simulink model "EEBL_Scenario_01_cs"  (Simulink 7.6)
settings: Solver=ode5  SolverMode=SingleTasking  StartTime=0.0  StopTime=inf  FixedStep=1/100  RelTol=1e-3
PreLoadFcn:
  | check_NUTS_defined;
  | 
  | assignin('base',['model_closed_' bdroot],false);addpath('../includes_V2x');
InitFcn:
  | PreScanExperimentInitFcn(bdroot)
StopFcn:
  | PreScanExperimentStopFcn(bdroot)
undefined symbols (not defined in the file or in its folder): acceleration, actorID, actorType, DiscIntNeverNeededParam, GPS_alt, GPS_lat, GPS_long, intmax, lightBarInUse, messageID, publicVehicleType, rotZ, sireneInUse, trafficLightPriority, turnAdvice, velocity, x_ini_VRML, y_ini_VRML, yawRate, z_ini_VRML
libraries: simulink x58, PreScanSimulinkLibrary x12, simulink_extras x10, PreScanUsefulBlocks x6, simulink_need_slupdate x1
(part 5 of 10)

== system EEBL_Scenario_01_cs/BMW_X5_1/Antenna_Rx_3_Demux ==
  AntennaR : Inport
  Bus Creator : BusCreator  Inputs=200
  Demux : Demux  Outputs=228
  Demux1 : Demux  Outputs=3
  Mux : Mux  Inputs=3
  Reorder : Subsystem  mask(Output reorder block){NrOfOutputs=228, NrOfObjects=2}
      mask prompts: NrOfOutputs "Number Of Outputs [-]"; NrOfObjects "Number Of Objects [-]"
      mask help: Change output order from object based to output type based
      mask init: same as EEBL_Scenario_01_cs/Audi_A8_1/Antenna_Rx_1_Demux/Reorder
  Terminator_{9..12,17..18,20..23,25..30} (16 alike) : Terminator
  compas converter : Subsystem
  xyz2GPS : PreScanUsefulBlocks/xyz2GPS  CoordinateCount=2  GPS_base=[0.000000 0.000000 0.000]
  Vehicle_ID : Outport
  GPS_pos_lat_[deg] : Outport  Port=2
  GPS_pos_long_[deg] : Outport  Port=3
  GPS_pos_alt_[m] : Outport  Port=4
  Velocity_[m/s] : Outport  Port=5
  Acceleration_[m/s2] : Outport  Port=6
  Heading [deg] : Outport  Port=7
  warning_signal_id : Outport  Port=8
  maneuvre_id : Outport  Port=9
  vehicle_type : Outport  Port=10
  brakingcapacity : Outport  Port=11
  vehicle_size : Outport  Port=12
  spare : Outport  Port=13
  wires:
  Bus Creator/1 -> spare/1
  compas converter/1(heading [deg]) -> Heading [deg]/1
  Demux/1 -> Vehicle_ID/1
  Demux/2 -> Terminator_9/1
  Demux/3 -> Terminator_10/1
  Demux/4 -> Terminator_11/1
  Demux/5 -> Terminator_12/1
  Demux/6 -> Mux/1  "pos_x"
  Demux/7 -> Mux/2  "pos_y"
  Demux/8 -> Mux/3  "pos_z"
  Demux/10 -> Terminator_17/1
  Demux/11 -> Terminator_18/1
  Demux/12 -> Acceleration_[m/s2]/1
  Demux/13 -> Terminator_20/1
  Demux/14 -> Terminator_21/1
  Demux/15 -> Terminator_22/1
  Demux/16 -> Terminator_23/1
  Demux/17 -> compas converter/1(rotz [rad])
  Demux/18 -> Terminator_25/1
  Demux/19 -> Terminator_26/1
  Demux/20 -> Terminator_27/1
  Demux/21 -> Terminator_28/1
  Demux/22 -> Terminator_29/1
  Demux/23 -> Terminator_30/1
  Demux/9 -> Velocity_[m/s]/1
  Demux/24 -> warning_signal_id/1
  Demux/25 -> maneuvre_id/1
  Demux/26 -> vehicle_type/1
  Demux/27 -> brakingcapacity/1
  Demux/28 -> vehicle_size/1
  xyz2GPS/1 -> Demux1/1
  Demux1/1 -> GPS_pos_lat_[deg]/1
  Demux1/2 -> GPS_pos_long_[deg]/1
  Demux1/3 -> GPS_pos_alt_[m]/1
  Mux/1 -> xyz2GPS/1
  Reorder/1(Out) -> Demux/1
  AntennaR/1 -> Reorder/1(In)
  Demux/29 -> Bus Creator/1  "warning"
  Demux/30 -> Bus Creator/2  "messageID"
  Demux/31 -> Bus Creator/3  "actorID"
  Demux/32 -> Bus Creator/4  "actorType"
  Demux/33 -> Bus Creator/5  "publicVehicleType"
  Demux/34 -> Bus Creator/6  "lightBarInUse"
  Demux/35 -> Bus Creator/7  "sireneInUse"
  Demux/36 -> Bus Creator/8  "velocity"
  Demux/37 -> Bus Creator/9  "acceleration"
  Demux/38 -> Bus Creator/10  "yawRate"
  Demux/39 -> Bus Creator/11  "turnAdvice"
  Demux/40 -> Bus Creator/12  "trafficLightPriority"
  Demux/41 -> Bus Creator/13  "GPS_lat"
  Demux/42 -> Bus Creator/14  "GPS_long"
  Demux/43 -> Bus Creator/15  "GPS_alt"
  Demux/44 -> Bus Creator/16  "rotZ"
  Demux/45 -> Bus Creator/17  "spare_17"
  Demux/46 -> Bus Creator/18  "spare_18"
  Demux/47 -> Bus Creator/19  "spare_19"
  Demux/48 -> Bus Creator/20  "spare_20"
  Demux/49 -> Bus Creator/21  "spare_21"
  Demux/50 -> Bus Creator/22  "spare_22"
  Demux/51 -> Bus Creator/23  "spare_23"
  Demux/52 -> Bus Creator/24  "spare_24"
  Demux/53 -> Bus Creator/25  "spare_25"
  Demux/54 -> Bus Creator/26  "spare_26"
  Demux/55 -> Bus Creator/27  "spare_27"
  Demux/56 -> Bus Creator/28  "spare_28"
  Demux/57 -> Bus Creator/29  "spare_29"
  Demux/58 -> Bus Creator/30  "spare_30"
  Demux/59 -> Bus Creator/31  "spare_31"
  Demux/60 -> Bus Creator/32  "spare_32"
  Demux/61 -> Bus Creator/33  "spare_33"
  Demux/62 -> Bus Creator/34  "spare_34"
  Demux/63 -> Bus Creator/35  "spare_35"
  Demux/64 -> Bus Creator/36  "spare_36"
  Demux/65 -> Bus Creator/37  "spare_37"
  Demux/66 -> Bus Creator/38  "spare_38"
  Demux/67 -> Bus Creator/39  "spare_39"
  Demux/68 -> Bus Creator/40  "spare_40"
  Demux/69 -> Bus Creator/41  "spare_41"
  Demux/70 -> Bus Creator/42  "spare_42"
  Demux/71 -> Bus Creator/43  "spare_43"
  Demux/72 -> Bus Creator/44  "spare_44"
  Demux/73 -> Bus Creator/45  "spare_45"
  Demux/74 -> Bus Creator/46  "spare_46"
  Demux/75 -> Bus Creator/47  "spare_47"
  Demux/76 -> Bus Creator/48  "spare_48"
  Demux/77 -> Bus Creator/49  "spare_49"
  Demux/78 -> Bus Creator/50  "spare_50"
  Demux/79 -> Bus Creator/51  "spare_51"
  Demux/80 -> Bus Creator/52  "spare_52"
  Demux/81 -> Bus Creator/53  "spare_53"
  Demux/82 -> Bus Creator/54  "spare_54"
  Demux/83 -> Bus Creator/55  "spare_55"
  Demux/84 -> Bus Creator/56  "spare_56"
  Demux/85 -> Bus Creator/57  "spare_57"
  Demux/86 -> Bus Creator/58  "spare_58"
  Demux/87 -> Bus Creator/59  "spare_59"
  Demux/88 -> Bus Creator/60  "spare_60"
  Demux/89 -> Bus Creator/61  "spare_61"
  Demux/90 -> Bus Creator/62  "spare_62"
  Demux/91 -> Bus Creator/63  "spare_63"
  Demux/92 -> Bus Creator/64  "spare_64"
  Demux/93 -> Bus Creator/65  "spare_65"
  Demux/94 -> Bus Creator/66  "spare_66"
  Demux/95 -> Bus Creator/67  "spare_67"
  Demux/96 -> Bus Creator/68  "spare_68"
  Demux/97 -> Bus Creator/69  "spare_69"
  Demux/98 -> Bus Creator/70  "spare_70"
  Demux/99 -> Bus Creator/71  "spare_71"
  Demux/100 -> Bus Creator/72  "spare_72"
  Demux/101 -> Bus Creator/73  "spare_73"
  Demux/102 -> Bus Creator/74  "spare_74"
  Demux/103 -> Bus Creator/75  "spare_75"
  Demux/104 -> Bus Creator/76  "spare_76"
  Demux/105 -> Bus Creator/77  "spare_77"
  Demux/106 -> Bus Creator/78  "spare_78"
  Demux/107 -> Bus Creator/79  "spare_79"
  Demux/108 -> Bus Creator/80  "spare_80"
  Demux/109 -> Bus Creator/81  "spare_81"
  Demux/110 -> Bus Creator/82  "spare_82"
  Demux/111 -> Bus Creator/83  "spare_83"
  Demux/112 -> Bus Creator/84  "spare_84"
  Demux/113 -> Bus Creator/85  "spare_85"
  Demux/114 -> Bus Creator/86  "spare_86"
  Demux/115 -> Bus Creator/87  "spare_87"
  Demux/116 -> Bus Creator/88  "spare_88"
  Demux/117 -> Bus Creator/89  "spare_89"
  Demux/118 -> Bus Creator/90  "spare_90"
  Demux/119 -> Bus Creator/91  "spare_91"
  Demux/120 -> Bus Creator/92  "spare_92"
  Demux/121 -> Bus Creator/93  "spare_93"
  Demux/122 -> Bus Creator/94  "spare_94"
  Demux/123 -> Bus Creator/95  "spare_95"
  Demux/124 -> Bus Creator/96  "spare_96"
  Demux/125 -> Bus Creator/97  "spare_97"
  Demux/126 -> Bus Creator/98  "spare_98"
  Demux/127 -> Bus Creator/99  "spare_99"
  Demux/128 -> Bus Creator/100  "spare_100"
  Demux/129 -> Bus Creator/101  "spare_101"
  Demux/130 -> Bus Creator/102  "spare_102"
  Demux/131 -> Bus Creator/103  "spare_103"
  Demux/132 -> Bus Creator/104  "spare_104"
  Demux/133 -> Bus Creator/105  "spare_105"
  Demux/134 -> Bus Creator/106  "spare_106"
  Demux/135 -> Bus Creator/107  "spare_107"
  Demux/136 -> Bus Creator/108  "spare_108"
  Demux/137 -> Bus Creator/109  "spare_109"
  Demux/138 -> Bus Creator/110  "spare_110"
  Demux/139 -> Bus Creator/111  "spare_111"
  Demux/140 -> Bus Creator/112  "spare_112"
  Demux/141 -> Bus Creator/113  "spare_113"
  Demux/142 -> Bus Creator/114  "spare_114"
  Demux/143 -> Bus Creator/115  "spare_115"
  Demux/144 -> Bus Creator/116  "spare_116"
  Demux/145 -> Bus Creator/117  "spare_117"
  Demux/146 -> Bus Creator/118  "spare_118"
  Demux/147 -> Bus Creator/119  "spare_119"
  Demux/148 -> Bus Creator/120  "spare_120"
  Demux/149 -> Bus Creator/121  "spare_121"
  Demux/150 -> Bus Creator/122  "spare_122"
  Demux/151 -> Bus Creator/123  "spare_123"
  Demux/152 -> Bus Creator/124  "spare_124"
  Demux/153 -> Bus Creator/125  "spare_125"
  Demux/154 -> Bus Creator/126  "spare_126"
  Demux/155 -> Bus Creator/127  "spare_127"
  Demux/156 -> Bus Creator/128  "spare_128"
  Demux/157 -> Bus Creator/129  "spare_129"
  Demux/158 -> Bus Creator/130  "spare_130"
  Demux/159 -> Bus Creator/131  "spare_131"
  Demux/160 -> Bus Creator/132  "spare_132"
  Demux/161 -> Bus Creator/133  "spare_133"
  Demux/162 -> Bus Creator/134  "spare_134"
  Demux/163 -> Bus Creator/135  "spare_135"
  Demux/164 -> Bus Creator/136  "spare_136"
  Demux/165 -> Bus Creator/137  "spare_137"
  Demux/166 -> Bus Creator/138  "spare_138"
  Demux/167 -> Bus Creator/139  "spare_139"
  Demux/168 -> Bus Creator/140  "spare_140"
  Demux/169 -> Bus Creator/141  "spare_141"
  Demux/170 -> Bus Creator/142  "spare_142"
  Demux/171 -> Bus Creator/143  "spare_143"
  Demux/172 -> Bus Creator/144  "spare_144"
  Demux/173 -> Bus Creator/145  "spare_145"
  Demux/174 -> Bus Creator/146  "spare_146"
  Demux/175 -> Bus Creator/147  "spare_147"
  Demux/176 -> Bus Creator/148  "spare_148"
  Demux/177 -> Bus Creator/149  "spare_149"
  Demux/178 -> Bus Creator/150  "spare_150"
  Demux/179 -> Bus Creator/151  "spare_151"
  Demux/180 -> Bus Creator/152  "spare_152"
  Demux/181 -> Bus Creator/153  "spare_153"
  Demux/182 -> Bus Creator/154  "spare_154"
  Demux/183 -> Bus Creator/155  "spare_155"
  Demux/184 -> Bus Creator/156  "spare_156"
  Demux/185 -> Bus Creator/157  "spare_157"
  Demux/186 -> Bus Creator/158  "spare_158"
  Demux/187 -> Bus Creator/159  "spare_159"
  Demux/188 -> Bus Creator/160  "spare_160"
  Demux/189 -> Bus Creator/161  "spare_161"
  Demux/190 -> Bus Creator/162  "spare_162"
  Demux/191 -> Bus Creator/163  "spare_163"
  Demux/192 -> Bus Creator/164  "spare_164"
  Demux/193 -> Bus Creator/165  "spare_165"
  Demux/194 -> Bus Creator/166  "spare_166"
  Demux/195 -> Bus Creator/167  "spare_167"
  Demux/196 -> Bus Creator/168  "spare_168"
  Demux/197 -> Bus Creator/169  "spare_169"
  Demux/198 -> Bus Creator/170  "spare_170"
  Demux/199 -> Bus Creator/171  "spare_171"
  Demux/200 -> Bus Creator/172  "spare_172"
  Demux/201 -> Bus Creator/173  "spare_173"
  Demux/202 -> Bus Creator/174  "spare_174"
  Demux/203 -> Bus Creator/175  "spare_175"
  Demux/204 -> Bus Creator/176  "spare_176"
  Demux/205 -> Bus Creator/177  "spare_177"
  Demux/206 -> Bus Creator/178  "spare_178"
  Demux/207 -> Bus Creator/179  "spare_179"
  Demux/208 -> Bus Creator/180  "spare_180"
  Demux/209 -> Bus Creator/181  "spare_181"
  Demux/210 -> Bus Creator/182  "spare_182"
  Demux/211 -> Bus Creator/183  "spare_183"
  Demux/212 -> Bus Creator/184  "spare_184"
  Demux/213 -> Bus Creator/185  "spare_185"
  Demux/214 -> Bus Creator/186  "spare_186"
  Demux/215 -> Bus Creator/187  "spare_187"
  Demux/216 -> Bus Creator/188  "spare_188"
  Demux/217 -> Bus Creator/189  "spare_189"
  Demux/218 -> Bus Creator/190  "spare_190"
  Demux/219 -> Bus Creator/191  "spare_191"
  Demux/220 -> Bus Creator/192  "spare_192"
  Demux/221 -> Bus Creator/193  "spare_193"
  Demux/222 -> Bus Creator/194  "spare_194"
  Demux/223 -> Bus Creator/195  "spare_195"
  Demux/224 -> Bus Creator/196  "spare_196"
  Demux/225 -> Bus Creator/197  "spare_197"
  Demux/226 -> Bus Creator/198  "spare_198"
  Demux/227 -> Bus Creator/199  "spare_199"
  Demux/228 -> Bus Creator/200  "spare_200"

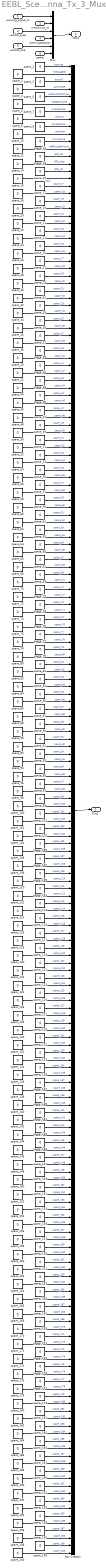
== system EEBL_Scenario_01_cs/BMW_X5_1/Antenna_Tx_3_Mux ==
  warning_signal_id : Inport  SampleTime=TimeStep
  maneuvre_id : Inport  Port=2  SampleTime=TimeStep
  vehicle_type : Inport  Port=3  SampleTime=TimeStep
  brakingcapacity : Inport  Port=4  SampleTime=TimeStep
  vehicle_size : Inport  Port=5  SampleTime=TimeStep
  spare : Inport  Port=6  SampleTime=TimeStep
  Bus Creator : BusCreator  Inputs=200
  Mux : Mux  Inputs=6
  spare_{1..200} (200 alike) : Constant  Value=0  SampleTime=TimeStep
  Out1 : Outport
  Out2 : Outport  Port=2  SampleTime=TimeStep
  wires:
  spare_200/1 -> Bus Creator/200  "spare_200"
  spare_199/1 -> Bus Creator/199  "spare_199"
  spare_198/1 -> Bus Creator/198  "spare_198"
  spare_197/1 -> Bus Creator/197  "spare_197"
  spare_196/1 -> Bus Creator/196  "spare_196"
  spare_195/1 -> Bus Creator/195  "spare_195"
  spare_194/1 -> Bus Creator/194  "spare_194"
  spare_193/1 -> Bus Creator/193  "spare_193"
  spare_192/1 -> Bus Creator/192  "spare_192"
  spare_191/1 -> Bus Creator/191  "spare_191"
  spare_190/1 -> Bus Creator/190  "spare_190"
  spare_189/1 -> Bus Creator/189  "spare_189"
  spare_188/1 -> Bus Creator/188  "spare_188"
  spare_187/1 -> Bus Creator/187  "spare_187"
  spare_186/1 -> Bus Creator/186  "spare_186"
  spare_185/1 -> Bus Creator/185  "spare_185"
  spare_184/1 -> Bus Creator/184  "spare_184"
  spare_183/1 -> Bus Creator/183  "spare_183"
  spare_182/1 -> Bus Creator/182  "spare_182"
  spare_181/1 -> Bus Creator/181  "spare_181"
  spare_180/1 -> Bus Creator/180  "spare_180"
  spare_179/1 -> Bus Creator/179  "spare_179"
  spare_178/1 -> Bus Creator/178  "spare_178"
  spare_177/1 -> Bus Creator/177  "spare_177"
  spare_176/1 -> Bus Creator/176  "spare_176"
  spare_175/1 -> Bus Creator/175  "spare_175"
  spare_174/1 -> Bus Creator/174  "spare_174"
  spare_173/1 -> Bus Creator/173  "spare_173"
  spare_172/1 -> Bus Creator/172  "spare_172"
  spare_171/1 -> Bus Creator/171  "spare_171"
  spare_170/1 -> Bus Creator/170  "spare_170"
  spare_169/1 -> Bus Creator/169  "spare_169"
  spare_168/1 -> Bus Creator/168  "spare_168"
  spare_167/1 -> Bus Creator/167  "spare_167"
  spare_166/1 -> Bus Creator/166  "spare_166"
  spare_165/1 -> Bus Creator/165  "spare_165"
  spare_164/1 -> Bus Creator/164  "spare_164"
  spare_163/1 -> Bus Creator/163  "spare_163"
  spare_162/1 -> Bus Creator/162  "spare_162"
  spare_161/1 -> Bus Creator/161  "spare_161"
  spare_160/1 -> Bus Creator/160  "spare_160"
  spare_159/1 -> Bus Creator/159  "spare_159"
  spare_158/1 -> Bus Creator/158  "spare_158"
  spare_157/1 -> Bus Creator/157  "spare_157"
  spare_156/1 -> Bus Creator/156  "spare_156"
  spare_155/1 -> Bus Creator/155  "spare_155"
  spare_154/1 -> Bus Creator/154  "spare_154"
  spare_153/1 -> Bus Creator/153  "spare_153"
  spare_152/1 -> Bus Creator/152  "spare_152"
  spare_151/1 -> Bus Creator/151  "spare_151"
  spare_150/1 -> Bus Creator/150  "spare_150"
  spare_149/1 -> Bus Creator/149  "spare_149"
  spare_148/1 -> Bus Creator/148  "spare_148"
  spare_147/1 -> Bus Creator/147  "spare_147"
  spare_146/1 -> Bus Creator/146  "spare_146"
  spare_145/1 -> Bus Creator/145  "spare_145"
  spare_144/1 -> Bus Creator/144  "spare_144"
  spare_143/1 -> Bus Creator/143  "spare_143"
  spare_142/1 -> Bus Creator/142  "spare_142"
  spare_141/1 -> Bus Creator/141  "spare_141"
  spare_140/1 -> Bus Creator/140  "spare_140"
  spare_139/1 -> Bus Creator/139  "spare_139"
  spare_138/1 -> Bus Creator/138  "spare_138"
  spare_137/1 -> Bus Creator/137  "spare_137"
  spare_136/1 -> Bus Creator/136  "spare_136"
  spare_135/1 -> Bus Creator/135  "spare_135"
  spare_134/1 -> Bus Creator/134  "spare_134"
  spare_133/1 -> Bus Creator/133  "spare_133"
  spare_132/1 -> Bus Creator/132  "spare_132"
  spare_131/1 -> Bus Creator/131  "spare_131"
  spare_130/1 -> Bus Creator/130  "spare_130"
  spare_129/1 -> Bus Creator/129  "spare_129"
  spare_128/1 -> Bus Creator/128  "spare_128"
  spare_127/1 -> Bus Creator/127  "spare_127"
  spare_126/1 -> Bus Creator/126  "spare_126"
  spare_125/1 -> Bus Creator/125  "spare_125"
  spare_124/1 -> Bus Creator/124  "spare_124"
  spare_123/1 -> Bus Creator/123  "spare_123"
  spare_122/1 -> Bus Creator/122  "spare_122"
  spare_121/1 -> Bus Creator/121  "spare_121"
  spare_120/1 -> Bus Creator/120  "spare_120"
  spare_119/1 -> Bus Creator/119  "spare_119"
  spare_118/1 -> Bus Creator/118  "spare_118"
  spare_117/1 -> Bus Creator/117  "spare_117"
  spare_116/1 -> Bus Creator/116  "spare_116"
  spare_115/1 -> Bus Creator/115  "spare_115"
  spare_114/1 -> Bus Creator/114  "spare_114"
  spare_113/1 -> Bus Creator/113  "spare_113"
  spare_112/1 -> Bus Creator/112  "spare_112"
  spare_111/1 -> Bus Creator/111  "spare_111"
  spare_110/1 -> Bus Creator/110  "spare_110"
  spare_109/1 -> Bus Creator/109  "spare_109"
  spare_108/1 -> Bus Creator/108  "spare_108"
  spare_107/1 -> Bus Creator/107  "spare_107"
  spare_106/1 -> Bus Creator/106  "spare_106"
  spare_105/1 -> Bus Creator/105  "spare_105"
  spare_104/1 -> Bus Creator/104  "spare_104"
  spare_103/1 -> Bus Creator/103  "spare_103"
  spare_102/1 -> Bus Creator/102  "spare_102"
  spare_101/1 -> Bus Creator/101  "spare_101"
  spare_100/1 -> Bus Creator/100  "spare_100"
  spare_99/1 -> Bus Creator/99  "spare_99"
  spare_98/1 -> Bus Creator/98  "spare_98"
  spare_97/1 -> Bus Creator/97  "spare_97"
  spare_96/1 -> Bus Creator/96  "spare_96"
  spare_95/1 -> Bus Creator/95  "spare_95"
  spare_94/1 -> Bus Creator/94  "spare_94"
  spare_93/1 -> Bus Creator/93  "spare_93"
  spare_92/1 -> Bus Creator/92  "spare_92"
  spare_91/1 -> Bus Creator/91  "spare_91"
  spare_90/1 -> Bus Creator/90  "spare_90"
  spare_89/1 -> Bus Creator/89  "spare_89"
  spare_88/1 -> Bus Creator/88  "spare_88"
  spare_87/1 -> Bus Creator/87  "spare_87"
  spare_86/1 -> Bus Creator/86  "spare_86"
  spare_85/1 -> Bus Creator/85  "spare_85"
  spare_84/1 -> Bus Creator/84  "spare_84"
  spare_83/1 -> Bus Creator/83  "spare_83"
  spare_82/1 -> Bus Creator/82  "spare_82"
  spare_81/1 -> Bus Creator/81  "spare_81"
  spare_80/1 -> Bus Creator/80  "spare_80"
  spare_79/1 -> Bus Creator/79  "spare_79"
  spare_78/1 -> Bus Creator/78  "spare_78"
  spare_77/1 -> Bus Creator/77  "spare_77"
  spare_76/1 -> Bus Creator/76  "spare_76"
  spare_75/1 -> Bus Creator/75  "spare_75"
  spare_74/1 -> Bus Creator/74  "spare_74"
  spare_73/1 -> Bus Creator/73  "spare_73"
  spare_72/1 -> Bus Creator/72  "spare_72"
  spare_71/1 -> Bus Creator/71  "spare_71"
  spare_70/1 -> Bus Creator/70  "spare_70"
  spare_69/1 -> Bus Creator/69  "spare_69"
  spare_68/1 -> Bus Creator/68  "spare_68"
  spare_67/1 -> Bus Creator/67  "spare_67"
  spare_66/1 -> Bus Creator/66  "spare_66"
  spare_65/1 -> Bus Creator/65  "spare_65"
  spare_64/1 -> Bus Creator/64  "spare_64"
  spare_63/1 -> Bus Creator/63  "spare_63"
  spare_62/1 -> Bus Creator/62  "spare_62"
  spare_61/1 -> Bus Creator/61  "spare_61"
  spare_60/1 -> Bus Creator/60  "spare_60"
  spare_59/1 -> Bus Creator/59  "spare_59"
  spare_58/1 -> Bus Creator/58  "spare_58"
  spare_57/1 -> Bus Creator/57  "spare_57"
  spare_56/1 -> Bus Creator/56  "spare_56"
  spare_55/1 -> Bus Creator/55  "spare_55"
  spare_54/1 -> Bus Creator/54  "spare_54"
  spare_53/1 -> Bus Creator/53  "spare_53"
  spare_52/1 -> Bus Creator/52  "spare_52"
  spare_51/1 -> Bus Creator/51  "spare_51"
  spare_50/1 -> Bus Creator/50  "spare_50"
  spare_49/1 -> Bus Creator/49  "spare_49"
  spare_48/1 -> Bus Creator/48  "spare_48"
  spare_47/1 -> Bus Creator/47  "spare_47"
  spare_46/1 -> Bus Creator/46  "spare_46"
  spare_45/1 -> Bus Creator/45  "spare_45"
  spare_44/1 -> Bus Creator/44  "spare_44"
  spare_43/1 -> Bus Creator/43  "spare_43"
  spare_42/1 -> Bus Creator/42  "spare_42"
  spare_41/1 -> Bus Creator/41  "spare_41"
  spare_40/1 -> Bus Creator/40  "spare_40"
  spare_39/1 -> Bus Creator/39  "spare_39"
  spare_38/1 -> Bus Creator/38  "spare_38"
  spare_37/1 -> Bus Creator/37  "spare_37"
  spare_36/1 -> Bus Creator/36  "spare_36"
  spare_35/1 -> Bus Creator/35  "spare_35"
  spare_34/1 -> Bus Creator/34  "spare_34"
  spare_33/1 -> Bus Creator/33  "spare_33"
  spare_32/1 -> Bus Creator/32  "spare_32"
  spare_31/1 -> Bus Creator/31  "spare_31"
  spare_30/1 -> Bus Creator/30  "spare_30"
  spare_29/1 -> Bus Creator/29  "spare_29"
  spare_28/1 -> Bus Creator/28  "spare_28"
  spare_27/1 -> Bus Creator/27  "spare_27"
  spare_26/1 -> Bus Creator/26  "spare_26"
  spare_25/1 -> Bus Creator/25  "spare_25"
  spare_24/1 -> Bus Creator/24  "spare_24"
  spare_23/1 -> Bus Creator/23  "spare_23"
  spare_22/1 -> Bus Creator/22  "spare_22"
  spare_21/1 -> Bus Creator/21  "spare_21"
  spare_19/1 -> Bus Creator/19  "spare_19"
  spare_18/1 -> Bus Creator/18  "spare_18"
  spare_17/1 -> Bus Creator/17  "spare_17"
  warning_signal_id/1 -> Mux/1
  maneuvre_id/1 -> Mux/2
  vehicle_type/1 -> Mux/3
  brakingcapacity/1 -> Mux/4
  vehicle_size/1 -> Mux/5
  Mux/1 -> Out1/1
  Bus Creator/1 -> Out2/1
  spare/1 -> Mux/6
  spare_1/1 -> Bus Creator/1  "warning"
  spare_2/1 -> Bus Creator/2  "messageID"
  spare_3/1 -> Bus Creator/3  "actorID"
  spare_4/1 -> Bus Creator/4  "actorType"
  spare_5/1 -> Bus Creator/5  "publicVehicleType"
  spare_6/1 -> Bus Creator/6  "lightBarInUse"
  spare_7/1 -> Bus Creator/7  "sireneInUse"
  spare_8/1 -> Bus Creator/8  "velocity"
  spare_9/1 -> Bus Creator/9  "acceleration"
  spare_10/1 -> Bus Creator/10  "yawRate"
  spare_11/1 -> Bus Creator/11  "turnAdvice"
  spare_12/1 -> Bus Creator/12  "trafficLightPriority"
  spare_13/1 -> Bus Creator/13  "GPS_lat"
  spare_14/1 -> Bus Creator/14  "GPS_long"
  spare_15/1 -> Bus Creator/15  "GPS_alt"
  spare_16/1 -> Bus Creator/16  "rotZ"
  spare_20/1 -> Bus Creator/20  "spare_20"

== system EEBL_Scenario_01_cs/BMW_X5_1/SELF_Demux ==
  SELF : Inport
  Demux1 : Demux  Outputs=3
  Demux2 : Demux  Outputs=3
  Demux3 : Demux  Outputs=[3 3 1 1]
  Demux4 : Demux  Outputs=3
  Gain : Gain  Gain=180/pi
  Gain1 : Gain  Gain=180/pi
  Selector : Selector  InputPortWidth=3  IndexOptions=Index vector (dialog)  Indices=[3]  OutputSizes=1
  compas converter : Subsystem
  xyz2GPS : PreScanUsefulBlocks/xyz2GPS  CoordinateCount=1  GPS_base=[0.000000 0.000000 0.000]
  x [m] : Outport
  y [m] : Outport  Port=2
  z [m] : Outport  Port=3
  rotx [deg] : Outport  Port=4
  roty [deg] : Outport  Port=5
  rotz [deg] : Outport  Port=6
  GPS lat [deg] : Outport  Port=7
  GPS long [deg] : Outport  Port=8
  GPS alt [m] : Outport  Port=9
  velocity [m/s] : Outport  Port=10
  heading [deg] : Outport  Port=11
  yaw rate [deg/s] : Outport  Port=12
  wires:
  Demux3/4 -> Gain1/1
  Gain1/1 -> yaw rate [deg/s]/1
  Demux3/3 -> velocity [m/s]/1
  compas converter/1(heading [deg]) -> heading [deg]/1
  xyz2GPS/1 -> Demux4/1
  Demux4/3 -> GPS alt [m]/1
  Demux4/2 -> GPS long [deg]/1
  Demux4/1 -> GPS lat [deg]/1
  Demux3/2 -> Gain/1, Selector/1
  Demux3/1 -> xyz2GPS/1, Demux1/1
  SELF/1 -> Demux3/1
  Demux2/3 -> rotz [deg]/1
  Demux2/2 -> roty [deg]/1
  Demux2/1 -> rotx [deg]/1
  Demux1/3 -> z [m]/1
  Demux1/2 -> y [m]/1
  Demux1/1 -> x [m]/1
  Gain/1 -> Demux2/1
  Selector/1 -> compas converter/1(rotz [rad])

== system EEBL_Scenario_01_cs/BMW_X5_1/Stop_sim ==
  Velocity : Inport
  Clock : Clock
      settings: Decimation=10
  Compare To Constant : simulink/Logic and Bit Operations/Compare To Constant  SystemSampleTime=-1  relop=>=  const=3.0  LogicOutDataTypeMode=uint8  ZeroCross=off
  Compare To Zero : simulink/Logic and Bit Operations/Compare To Zero  SystemSampleTime=-1  relop=<=  LogicOutDataTypeMode=boolean
  Logical Operator : Logic  AllPortsSameDT=off  OutDataTypeStr=boolean
  Stop Simulation : Stop
  wires:
  Clock/1 -> Compare To Constant/1
  Compare To Zero/1 -> Logical Operator/1
  Compare To Constant/1 -> Logical Operator/2
  Logical Operator/1 -> Stop Simulation/1
  Velocity/1 -> Compare To Zero/1

== system EEBL_Scenario_01_cs/BMW_X5_1/Trajectories ==
  DISPLAY : M-S-Function  FunctionName=msfcn_EEB_Scenario_01
  ElapsedTrack1 : Subsystem  Tag=ElapsedTrack  mask(PreScan Demux Block:){Filename='Trajectory_2_Path.mat'}
      mask prompts: Filename "Name path-file"
      mask init:
      | route=load(['trajectories/',Filename]);
      | 
      | s=route.path(1,:);
      | x=route.path(2,:);
      | y=route.path(3,:);
      | z=route.path(4,:);
      | roll=route.path(5,:);
      | pitch=route.path(6,:);
      | yaw=route.path(7,:);
      settings: DeleteFcn=PreScanBlockDeleteFcn;
  Integrator : Integrator  LimitOutput=on  UpperSaturationLimit=24  LowerSaturationLimit=0
  Integrator1 : DiscreteIntegrator  Tag=TrajIntegrator  SampleTime=1/100  ICPrevOutput=DiscIntNeverNeededParam  ICPrevScaledInput=DiscIntNeverNeededParam
  Selector1 : Constant  Tag=TrajSubSelector  Value=2
  Sum : Sum  Inputs=|+-
  Traj2State1 : Subsystem  Tag=Traj2State
      settings: DeleteFcn=PreScanBlockDeleteFcn;
      mask Type: PreScan Demux Block:
  TrajSwitch1 : MultiPortSwitch  Tag=TrajSubSwitch  Inputs=2  zeroidx=off
  Trajectory_2 : Subsystem  Tag=Trajectory  mask(PreScan Source Block: Trajectory){FileName='Trajectory_2.mat', TimeStep=1/100}
      mask prompts: TimeStep "Time Step [s]"
      mask help:
      | The Trajectory block contains the trajectories defined in the PreScan Experiment Editor. The output of the trajectory block is the (vehicle) State.
      |
      | For more information, please click Help.
      mask init: same as EEBL_Scenario_01_cs/Audi_A8_1/Trajectories/Trajectory_1
      settings: DeleteFcn=PreScanBlockDeleteFcn;
      mask Help: eval('openHelp(312)')
      mask Display: fprintf(FileName)
  Trajectory_2_Offset : Constant  Tag=TrajectoryOffset  Value="[0  0  0  0  0  0]"
  Velocity1 : Constant  Tag=TrajVelocity  Value=24
  State : Outport  Tag=TrajOutport
  wires:
  DISPLAY/1 -> Integrator/1
  Integrator/1 -> Sum/2
  Trajectory_2/1(trajectory) -> Traj2State1/1(Traj Org)
  Trajectory_2_Offset/1 -> Traj2State1/2(Offset), ElapsedTrack1/1(Offset)
  Integrator1/1 -> ElapsedTrack1/2(s)
  Velocity1/1 -> Sum/1
  Selector1/1 -> TrajSwitch1/1
  Traj2State1/1(state) -> TrajSwitch1/2
  ElapsedTrack1/1(state) -> TrajSwitch1/3
  TrajSwitch1/1 -> State/1
  Sum/1 -> Integrator1/1

== system EEBL_Scenario_01_cs/BMW_X5_1/VISULightSource_Mux ==
  IndicatorLightsLeft : Inport
  IndicatorLightsRight : Inport  Port=2
  FogLightRearLeft : Inport  Port=3
  FogLightRearRight : Inport  Port=4
  FogLightFrontLeft : Inport  Port=5
  FogLightFrontRight : Inport  Port=6
  MainLightRearLeft : Inport  Port=7
  MainLightRearRight : Inport  Port=8
  MainLightFrontLeft : Inport  Port=9
  MainLightFrontRight : Inport  Port=10
  BrakeLightLeft : Inport  Port=11
  BrakeLightRight : Inport  Port=12
  SubMuxLightSource : Mux  Inputs=12
  Lights : Outport
  wires:
  SubMuxLightSource/1 -> Lights/1
  IndicatorLightsLeft/1 -> SubMuxLightSource/1
  IndicatorLightsRight/1 -> SubMuxLightSource/2
  FogLightRearLeft/1 -> SubMuxLightSource/3
  FogLightRearRight/1 -> SubMuxLightSource/4
  FogLightFrontLeft/1 -> SubMuxLightSource/5
  FogLightFrontRight/1 -> SubMuxLightSource/6
  MainLightRearLeft/1 -> SubMuxLightSource/7
  MainLightRearRight/1 -> SubMuxLightSource/8
  MainLightFrontLeft/1 -> SubMuxLightSource/9
  MainLightFrontRight/1 -> SubMuxLightSource/10
  BrakeLightLeft/1 -> SubMuxLightSource/11
  BrakeLightRight/1 -> SubMuxLightSource/12

== system EEBL_Scenario_01_cs/BMW_X5_1/VISUSteer_Mux ==
  Column [deg] : Inport
  Steer [deg] : Inport  Port=2
  Mux2 : Mux  Inputs=2
  Steer : Outport
  wires:
  Column [deg]/1 -> Mux2/2
  Mux2/1 -> Steer/1
  Steer [deg]/1 -> Mux2/1

== system EEBL_Scenario_01_cs/BMW_X5_1/VISUWheels_Mux ==
  Steer Angle Front [deg] : Inport  SampleTime=TimeStep
  Steer Angle Rear [deg] : Inport  Port=2  SampleTime=TimeStep
  Velocity [m/s] : Inport  Port=3  SampleTime=TimeStep
  zDisp FL [m] : Inport  Port=4  SampleTime=TimeStep
  zDisp FR [m] : Inport  Port=5  SampleTime=TimeStep
  zDisp RL [m] : Inport  Port=6  SampleTime=TimeStep
  zDisp RR [m] : Inport  Port=7  SampleTime=TimeStep
  Constant{,1..3} (4 alike) : Constant  Value=[0 0]  SampleTime=TimeStep
  Constant{4..7} (4 alike) : Constant  Value=0  SampleTime=TimeStep
  Discrete-Time Integrator : DiscreteIntegrator  SampleTime=TimeStep  ICPrevOutput=DiscIntNeverNeededParam  ICPrevScaledInput=DiscIntNeverNeededParam
  Mux{,1..3} (4 alike) : Mux  Inputs=3
  Mux{4,6..8} (4 alike) : Mux  Inputs=[2 1]
  Mux5 : Mux  Inputs=[3 3 3 3 3 3 3 3]
  Radians to Degrees : simulink_extras/Transformations/Radians to Degrees  SystemSampleTime=-1
  omega=V/Rwheel : Gain  Gain=1/0.29
  Wheels : Outport
  wires:
  Mux7/1 -> Mux5/5  "xyz displacement RL [m]"
  Discrete-Time Integrator/1 -> Mux/2, Mux1/2, Mux2/2, Mux3/2  "roty"
  Radians to Degrees/1 -> Discrete-Time Integrator/1
  Constant7/1 -> Mux3/1  "rotx"
  Constant6/1 -> Mux2/1  "rotx"
  Constant5/1 -> Mux1/1  "rotx"
  Constant4/1 -> Mux/1  "rotx"
  Steer Angle Front [deg]/1 -> Mux1/3, Mux/3  "rotz"
  Steer Angle Rear [deg]/1 -> Mux3/3, Mux2/3  "rotz"
  Mux8/1 -> Mux5/7  "xyz displacement RR [m]"
  Mux6/1 -> Mux5/3  "xyz displacement FR [m]"
  Mux4/1 -> Mux5/1  "xyz displacement FL [m]"
  Constant3/1 -> Mux8/1
  Constant2/1 -> Mux7/1
  Constant1/1 -> Mux6/1
  Constant/1 -> Mux4/1
  zDisp RR [m]/1 -> Mux8/2
  zDisp RL [m]/1 -> Mux7/2
  zDisp FR [m]/1 -> Mux6/2
  zDisp FL [m]/1 -> Mux4/2
  Mux5/1 -> Wheels/1
  omega=V/Rwheel/1 -> Radians to Degrees/1  "rotational speed [rad/s]"
  Velocity [m/s]/1 -> omega=V/Rwheel/1
  Mux1/1 -> Mux5/4  "xyz rotation FR [deg]"
  Mux/1 -> Mux5/2  "xyz rotation FL [deg]"
  Mux3/1 -> Mux5/8  "xyz rotation RR [deg]"
  Mux2/1 -> Mux5/6  "xyz rotation RL [deg]"

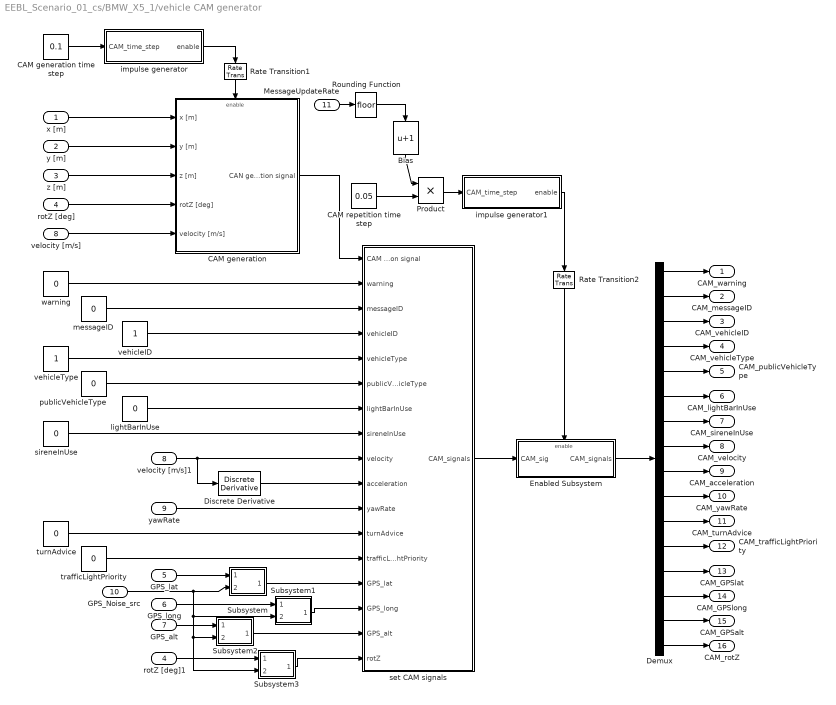
== system EEBL_Scenario_01_cs/BMW_X5_1/vehicle CAM generator ==
  x [m] : Inport
  y [m] : Inport  Port=2
  z [m] : Inport  Port=3
  rotZ [deg] : Inport  Port=4
  GPS_lat : Inport  Port=5
  GPS_long : Inport  Port=6
  GPS_alt : Inport  Port=7
  velocity [m/s] : Inport  Port=8
  yawRate : Inport  Port=9
  GPS_Noise_src : Inport  Port=10
  MessageUpdateRate : Inport  Port=11
  Bias : Bias  Bias=1
  CAM generation : Subsystem  TreatAsAtomicUnit=on
  CAM generation time step : Constant  Value=0.1
  CAM repetition time step : Constant  Value=0.05
  Demux : Demux  Outputs=16
  Discrete Derivative : simulink/Discrete/Discrete Derivative  SystemSampleTime=-1  gainval=1.0  ICPrevScaledInput=0.0  OutMin=[]  OutMax=[]  OutDataType=fixdt(1, 16)  OutScaling=2^-10  DoSatur=off
  Enabled Subsystem : Subsystem  TreatAsAtomicUnit=on
  Product : Product  RndMeth=Zero
  Rate Transition1 : RateTransition  Integrity=off  OutPortSampleTimeOpt=Inherit
  Rate Transition2 : RateTransition  Integrity=off  OutPortSampleTimeOpt=Inherit
  Rounding Function : Rounding
  Subsystem : Subsystem
  Subsystem1 : Subsystem
  Subsystem2 : Subsystem
  Subsystem3 : Subsystem
  impulse generator : Subsystem
  impulse generator1 : Subsystem
  lightBarInUse : Constant  Value=0
  messageID : Constant  Value=0
  publicVehicleType : Constant  Value=0
  rotZ [deg]1 : InportShadow  Port=4
  set CAM signals : Subsystem
  sireneInUse : Constant  Value=0
  trafficLightPriority : Constant  Value=0
  turnAdvice : Constant  Value=0
  vehicleID : Constant
  vehicleType : Constant
  velocity [m/s]1 : InportShadow  Port=8
  warning : Constant  Value=0
  CAM_warning : Outport
  CAM_messageID : Outport  Port=2
  CAM_vehicleID : Outport  Port=3
  CAM_vehicleType : Outport  Port=4
  CAM_publicVehicleType : Outport  Port=5
  CAM_lightBarInUse : Outport  Port=6
  CAM_sireneInUse : Outport  Port=7
  CAM_velocity : Outport  Port=8
  CAM_acceleration : Outport  Port=9
  CAM_yawRate : Outport  Port=10
  CAM_turnAdvice : Outport  Port=11
  CAM_trafficLightPriority : Outport  Port=12
  CAM_GPSlat : Outport  Port=13
  CAM_GPSlong : Outport  Port=14
  CAM_GPSalt : Outport  Port=15
  CAM_rotZ : Outport  Port=16
  wires:
  CAM generation time step/1 -> impulse generator/1(CAM_time_step)
  impulse generator1/1(enable) -> Rate Transition2/1
  warning/1 -> set CAM signals/2(warning)
  messageID/1 -> set CAM signals/3(messageID)
  vehicleID/1 -> set CAM signals/4(vehicleID)
  vehicleType/1 -> set CAM signals/5(vehicleType)
  publicVehicleType/1 -> set CAM signals/6(publicVehicleType)
  lightBarInUse/1 -> set CAM signals/7(lightBarInUse)
  sireneInUse/1 -> set CAM signals/8(sireneInUse)
  velocity [m/s]1/1 -> Discrete Derivative/1, set CAM signals/9(velocity)
  Discrete Derivative/1 -> set CAM signals/10(acceleration)
  yawRate/1 -> set CAM signals/11(yawRate)
  turnAdvice/1 -> set CAM signals/12(turnAdvice)
  trafficLightPriority/1 -> set CAM signals/13(trafficLightPriority)
  GPS_lat/1 -> Subsystem/1(In1)
  GPS_long/1 -> Subsystem1/1(In1)
  GPS_alt/1 -> Subsystem2/1(In1)
  rotZ [deg]1/1 -> Subsystem3/1(In1)
  CAM generation/1(CAN generation signal) -> set CAM signals/1(CAM generation signal)
  x [m]/1 -> CAM generation/1(x [m])
  y [m]/1 -> CAM generation/2(y [m])
  z [m]/1 -> CAM generation/3(z [m])
  rotZ [deg]/1 -> CAM generation/4(rotZ [deg])
  velocity [m/s]/1 -> CAM generation/5(velocity [m/s])
  impulse generator/1(enable) -> Rate Transition1/1
  Rate Transition1/1 -> CAM generation/Enable
  set CAM signals/1(CAM_signals) -> Enabled Subsystem/1(CAM_sig)
  Rate Transition2/1 -> Enabled Subsystem/Enable
  Enabled Subsystem/1(CAM_signals) -> Demux/1
  Demux/1 -> CAM_warning/1
  Demux/2 -> CAM_messageID/1
  Demux/3 -> CAM_vehicleID/1
  Demux/4 -> CAM_vehicleType/1
  Demux/5 -> CAM_publicVehicleType/1
  Demux/6 -> CAM_lightBarInUse/1
  Demux/7 -> CAM_sireneInUse/1
  Demux/8 -> CAM_velocity/1
  Demux/9 -> CAM_acceleration/1
  Demux/10 -> CAM_yawRate/1
  Demux/11 -> CAM_turnAdvice/1
  Demux/12 -> CAM_trafficLightPriority/1
  Demux/13 -> CAM_GPSlat/1
  Demux/14 -> CAM_GPSlong/1
  Demux/15 -> CAM_GPSalt/1
  Demux/16 -> CAM_rotZ/1
  Subsystem/1(Out1) -> set CAM signals/14(GPS_lat)
  Subsystem1/1(Out1) -> set CAM signals/15(GPS_long)
  Subsystem2/1(Out1) -> set CAM signals/16(GPS_alt)
  Subsystem3/1(Out1) -> set CAM signals/17(rotZ)
  Product/1 -> impulse generator1/1(CAM_time_step)
  CAM repetition time step/1 -> Product/2
  MessageUpdateRate/1 -> Rounding Function/1
  Rounding Function/1 -> Bias/1
  Bias/1 -> Product/1
  GPS_Noise_src/1 -> Subsystem/2(GPS_Noise_src), Subsystem1/2(GPS_Noise_src), Subsystem2/2(GPS_Noise_src), Subsystem3/2(GPS_Noise_src)

== system EEBL_Scenario_01_cs/CollisionDetection/retrieve CollisionDetection signal ==
  In : Inport
  Constant1 : Constant  Value=0
  Relational Operator : RelationalOperator  Operator=>  OutDataTypeStr=boolean
  Selector : Selector  InputPortWidth=10  IndexOptions=Index vector (dialog)  Indices=[1 3 5 7 9]  OutputSizes=1
  Out : Outport
  wires:
  Relational Operator/1 -> Out/1
  In/1 -> Selector/1
  Selector/1 -> Relational Operator/1
  Constant1/1 -> Relational Operator/2

== system EEBL_Scenario_01_cs/RectangularBox_1/Antenna_Rx_2_Demux ==
  AntennaR : Inport
  Bus Creator : BusCreator  Inputs=200
  Demux : Demux  Outputs=228
  Demux1 : Demux  Outputs=3
  Mux : Mux  Inputs=3
  Reorder : Subsystem  mask(Output reorder block){NrOfOutputs=228, NrOfObjects=2}
      mask prompts: NrOfOutputs "Number Of Outputs [-]"; NrOfObjects "Number Of Objects [-]"
      mask help: Change output order from object based to output type based
      mask init: same as EEBL_Scenario_01_cs/Audi_A8_1/Antenna_Rx_1_Demux/Reorder
  Terminator_{9..12,17..18,20..23,25..30} (16 alike) : Terminator
  compas converter : Subsystem
  xyz2GPS : PreScanUsefulBlocks/xyz2GPS  CoordinateCount=2  GPS_base=[0.000000 0.000000 0.000]
  Vehicle_ID : Outport
  GPS_pos_lat_[deg] : Outport  Port=2
  GPS_pos_long_[deg] : Outport  Port=3
  GPS_pos_alt_[m] : Outport  Port=4
  Velocity_[m/s] : Outport  Port=5
  Acceleration_[m/s2] : Outport  Port=6
  Heading [deg] : Outport  Port=7
  warning_signal_id : Outport  Port=8
  maneuvre_id : Outport  Port=9
  vehicle_type : Outport  Port=10
  brakingcapacity : Outport  Port=11
  vehicle_size : Outport  Port=12
  spare : Outport  Port=13
  wires:
  Bus Creator/1 -> spare/1
  compas converter/1(heading [deg]) -> Heading [deg]/1
  Demux/1 -> Vehicle_ID/1
  Demux/2 -> Terminator_9/1
  Demux/3 -> Terminator_10/1
  Demux/4 -> Terminator_11/1
  Demux/5 -> Terminator_12/1
  Demux/6 -> Mux/1  "pos_x"
  Demux/7 -> Mux/2  "pos_y"
  Demux/8 -> Mux/3  "pos_z"
  Demux/10 -> Terminator_17/1
  Demux/11 -> Terminator_18/1
  Demux/12 -> Acceleration_[m/s2]/1
  Demux/13 -> Terminator_20/1
  Demux/14 -> Terminator_21/1
  Demux/15 -> Terminator_22/1
  Demux/16 -> Terminator_23/1
  Demux/17 -> compas converter/1(rotz [rad])
  Demux/18 -> Terminator_25/1
  Demux/19 -> Terminator_26/1
  Demux/20 -> Terminator_27/1
  Demux/21 -> Terminator_28/1
  Demux/22 -> Terminator_29/1
  Demux/23 -> Terminator_30/1
  Demux/9 -> Velocity_[m/s]/1
  Demux/24 -> warning_signal_id/1
  Demux/25 -> maneuvre_id/1
  Demux/26 -> vehicle_type/1
  Demux/27 -> brakingcapacity/1
  Demux/28 -> vehicle_size/1
  xyz2GPS/1 -> Demux1/1
  Demux1/1 -> GPS_pos_lat_[deg]/1
  Demux1/2 -> GPS_pos_long_[deg]/1
  Demux1/3 -> GPS_pos_alt_[m]/1
  Mux/1 -> xyz2GPS/1
  Reorder/1(Out) -> Demux/1
  AntennaR/1 -> Reorder/1(In)
  Demux/29 -> Bus Creator/1  "warning"
  Demux/30 -> Bus Creator/2  "messageID"
  Demux/31 -> Bus Creator/3  "actorID"
  Demux/32 -> Bus Creator/4  "actorType"
  Demux/33 -> Bus Creator/5  "publicVehicleType"
  Demux/34 -> Bus Creator/6  "lightBarInUse"
  Demux/35 -> Bus Creator/7  "sireneInUse"
  Demux/36 -> Bus Creator/8  "velocity"
  Demux/37 -> Bus Creator/9  "acceleration"
  Demux/38 -> Bus Creator/10  "yawRate"
  Demux/39 -> Bus Creator/11  "turnAdvice"
  Demux/40 -> Bus Creator/12  "trafficLightPriority"
  Demux/41 -> Bus Creator/13  "GPS_lat"
  Demux/42 -> Bus Creator/14  "GPS_long"
  Demux/43 -> Bus Creator/15  "GPS_alt"
  Demux/44 -> Bus Creator/16  "rotZ"
  Demux/45 -> Bus Creator/17  "spare_17"
  Demux/46 -> Bus Creator/18  "spare_18"
  Demux/47 -> Bus Creator/19  "spare_19"
  Demux/48 -> Bus Creator/20  "spare_20"
  Demux/49 -> Bus Creator/21  "spare_21"
  Demux/50 -> Bus Creator/22  "spare_22"
  Demux/51 -> Bus Creator/23  "spare_23"
  Demux/52 -> Bus Creator/24  "spare_24"
  Demux/53 -> Bus Creator/25  "spare_25"
  Demux/54 -> Bus Creator/26  "spare_26"
  Demux/55 -> Bus Creator/27  "spare_27"
  Demux/56 -> Bus Creator/28  "spare_28"
  Demux/57 -> Bus Creator/29  "spare_29"
  Demux/58 -> Bus Creator/30  "spare_30"
  Demux/59 -> Bus Creator/31  "spare_31"
  Demux/60 -> Bus Creator/32  "spare_32"
  Demux/61 -> Bus Creator/33  "spare_33"
  Demux/62 -> Bus Creator/34  "spare_34"
  Demux/63 -> Bus Creator/35  "spare_35"
  Demux/64 -> Bus Creator/36  "spare_36"
  Demux/65 -> Bus Creator/37  "spare_37"
  Demux/66 -> Bus Creator/38  "spare_38"
  Demux/67 -> Bus Creator/39  "spare_39"
  Demux/68 -> Bus Creator/40  "spare_40"
  Demux/69 -> Bus Creator/41  "spare_41"
  Demux/70 -> Bus Creator/42  "spare_42"
  Demux/71 -> Bus Creator/43  "spare_43"
  Demux/72 -> Bus Creator/44  "spare_44"
  Demux/73 -> Bus Creator/45  "spare_45"
  Demux/74 -> Bus Creator/46  "spare_46"
  Demux/75 -> Bus Creator/47  "spare_47"
  Demux/76 -> Bus Creator/48  "spare_48"
  Demux/77 -> Bus Creator/49  "spare_49"
  Demux/78 -> Bus Creator/50  "spare_50"
  Demux/79 -> Bus Creator/51  "spare_51"
  Demux/80 -> Bus Creator/52  "spare_52"
  Demux/81 -> Bus Creator/53  "spare_53"
  Demux/82 -> Bus Creator/54  "spare_54"
  Demux/83 -> Bus Creator/55  "spare_55"
  Demux/84 -> Bus Creator/56  "spare_56"
  Demux/85 -> Bus Creator/57  "spare_57"
  Demux/86 -> Bus Creator/58  "spare_58"
  Demux/87 -> Bus Creator/59  "spare_59"
  Demux/88 -> Bus Creator/60  "spare_60"
  Demux/89 -> Bus Creator/61  "spare_61"
  Demux/90 -> Bus Creator/62  "spare_62"
  Demux/91 -> Bus Creator/63  "spare_63"
  Demux/92 -> Bus Creator/64  "spare_64"
  Demux/93 -> Bus Creator/65  "spare_65"
  Demux/94 -> Bus Creator/66  "spare_66"
  Demux/95 -> Bus Creator/67  "spare_67"
  Demux/96 -> Bus Creator/68  "spare_68"
  Demux/97 -> Bus Creator/69  "spare_69"
  Demux/98 -> Bus Creator/70  "spare_70"
  Demux/99 -> Bus Creator/71  "spare_71"
  Demux/100 -> Bus Creator/72  "spare_72"
  Demux/101 -> Bus Creator/73  "spare_73"
  Demux/102 -> Bus Creator/74  "spare_74"
  Demux/103 -> Bus Creator/75  "spare_75"
  Demux/104 -> Bus Creator/76  "spare_76"
  Demux/105 -> Bus Creator/77  "spare_77"
  Demux/106 -> Bus Creator/78  "spare_78"
  Demux/107 -> Bus Creator/79  "spare_79"
  Demux/108 -> Bus Creator/80  "spare_80"
  Demux/109 -> Bus Creator/81  "spare_81"
  Demux/110 -> Bus Creator/82  "spare_82"
  Demux/111 -> Bus Creator/83  "spare_83"
  Demux/112 -> Bus Creator/84  "spare_84"
  Demux/113 -> Bus Creator/85  "spare_85"
  Demux/114 -> Bus Creator/86  "spare_86"
  Demux/115 -> Bus Creator/87  "spare_87"
  Demux/116 -> Bus Creator/88  "spare_88"
  Demux/117 -> Bus Creator/89  "spare_89"
  Demux/118 -> Bus Creator/90  "spare_90"
  Demux/119 -> Bus Creator/91  "spare_91"
  Demux/120 -> Bus Creator/92  "spare_92"
  Demux/121 -> Bus Creator/93  "spare_93"
  Demux/122 -> Bus Creator/94  "spare_94"
  Demux/123 -> Bus Creator/95  "spare_95"
  Demux/124 -> Bus Creator/96  "spare_96"
  Demux/125 -> Bus Creator/97  "spare_97"
  Demux/126 -> Bus Creator/98  "spare_98"
  Demux/127 -> Bus Creator/99  "spare_99"
  Demux/128 -> Bus Creator/100  "spare_100"
  Demux/129 -> Bus Creator/101  "spare_101"
  Demux/130 -> Bus Creator/102  "spare_102"
  Demux/131 -> Bus Creator/103  "spare_103"
  Demux/132 -> Bus Creator/104  "spare_104"
  Demux/133 -> Bus Creator/105  "spare_105"
  Demux/134 -> Bus Creator/106  "spare_106"
  Demux/135 -> Bus Creator/107  "spare_107"
  Demux/136 -> Bus Creator/108  "spare_108"
  Demux/137 -> Bus Creator/109  "spare_109"
  Demux/138 -> Bus Creator/110  "spare_110"
  Demux/139 -> Bus Creator/111  "spare_111"
  Demux/140 -> Bus Creator/112  "spare_112"
  Demux/141 -> Bus Creator/113  "spare_113"
  Demux/142 -> Bus Creator/114  "spare_114"
  Demux/143 -> Bus Creator/115  "spare_115"
  Demux/144 -> Bus Creator/116  "spare_116"
  Demux/145 -> Bus Creator/117  "spare_117"
  Demux/146 -> Bus Creator/118  "spare_118"
  Demux/147 -> Bus Creator/119  "spare_119"
  Demux/148 -> Bus Creator/120  "spare_120"
  Demux/149 -> Bus Creator/121  "spare_121"
  Demux/150 -> Bus Creator/122  "spare_122"
  Demux/151 -> Bus Creator/123  "spare_123"
  Demux/152 -> Bus Creator/124  "spare_124"
  Demux/153 -> Bus Creator/125  "spare_125"
  Demux/154 -> Bus Creator/126  "spare_126"
  Demux/155 -> Bus Creator/127  "spare_127"
  Demux/156 -> Bus Creator/128  "spare_128"
  Demux/157 -> Bus Creator/129  "spare_129"
  Demux/158 -> Bus Creator/130  "spare_130"
  Demux/159 -> Bus Creator/131  "spare_131"
  Demux/160 -> Bus Creator/132  "spare_132"
  Demux/161 -> Bus Creator/133  "spare_133"
  Demux/162 -> Bus Creator/134  "spare_134"
  Demux/163 -> Bus Creator/135  "spare_135"
  Demux/164 -> Bus Creator/136  "spare_136"
  Demux/165 -> Bus Creator/137  "spare_137"
  Demux/166 -> Bus Creator/138  "spare_138"
  Demux/167 -> Bus Creator/139  "spare_139"
  Demux/168 -> Bus Creator/140  "spare_140"
  Demux/169 -> Bus Creator/141  "spare_141"
  Demux/170 -> Bus Creator/142  "spare_142"
  Demux/171 -> Bus Creator/143  "spare_143"
  Demux/172 -> Bus Creator/144  "spare_144"
  Demux/173 -> Bus Creator/145  "spare_145"
  Demux/174 -> Bus Creator/146  "spare_146"
  Demux/175 -> Bus Creator/147  "spare_147"
  Demux/176 -> Bus Creator/148  "spare_148"
  Demux/177 -> Bus Creator/149  "spare_149"
  Demux/178 -> Bus Creator/150  "spare_150"
  Demux/179 -> Bus Creator/151  "spare_151"
  Demux/180 -> Bus Creator/152  "spare_152"
  Demux/181 -> Bus Creator/153  "spare_153"
  Demux/182 -> Bus Creator/154  "spare_154"
  Demux/183 -> Bus Creator/155  "spare_155"
  Demux/184 -> Bus Creator/156  "spare_156"
  Demux/185 -> Bus Creator/157  "spare_157"
  Demux/186 -> Bus Creator/158  "spare_158"
  Demux/187 -> Bus Creator/159  "spare_159"
  Demux/188 -> Bus Creator/160  "spare_160"
  Demux/189 -> Bus Creator/161  "spare_161"
  Demux/190 -> Bus Creator/162  "spare_162"
  Demux/191 -> Bus Creator/163  "spare_163"
  Demux/192 -> Bus Creator/164  "spare_164"
  Demux/193 -> Bus Creator/165  "spare_165"
  Demux/194 -> Bus Creator/166  "spare_166"
  Demux/195 -> Bus Creator/167  "spare_167"
  Demux/196 -> Bus Creator/168  "spare_168"
  Demux/197 -> Bus Creator/169  "spare_169"
  Demux/198 -> Bus Creator/170  "spare_170"
  Demux/199 -> Bus Creator/171  "spare_171"
  Demux/200 -> Bus Creator/172  "spare_172"
  Demux/201 -> Bus Creator/173  "spare_173"
  Demux/202 -> Bus Creator/174  "spare_174"
  Demux/203 -> Bus Creator/175  "spare_175"
  Demux/204 -> Bus Creator/176  "spare_176"
  Demux/205 -> Bus Creator/177  "spare_177"
  Demux/206 -> Bus Creator/178  "spare_178"
  Demux/207 -> Bus Creator/179  "spare_179"
  Demux/208 -> Bus Creator/180  "spare_180"
  Demux/209 -> Bus Creator/181  "spare_181"
  Demux/210 -> Bus Creator/182  "spare_182"
  Demux/211 -> Bus Creator/183  "spare_183"
  Demux/212 -> Bus Creator/184  "spare_184"
  Demux/213 -> Bus Creator/185  "spare_185"
  Demux/214 -> Bus Creator/186  "spare_186"
  Demux/215 -> Bus Creator/187  "spare_187"
  Demux/216 -> Bus Creator/188  "spare_188"
  Demux/217 -> Bus Creator/189  "spare_189"
  Demux/218 -> Bus Creator/190  "spare_190"
  Demux/219 -> Bus Creator/191  "spare_191"
  Demux/220 -> Bus Creator/192  "spare_192"
  Demux/221 -> Bus Creator/193  "spare_193"
  Demux/222 -> Bus Creator/194  "spare_194"
  Demux/223 -> Bus Creator/195  "spare_195"
  Demux/224 -> Bus Creator/196  "spare_196"
  Demux/225 -> Bus Creator/197  "spare_197"
  Demux/226 -> Bus Creator/198  "spare_198"
  Demux/227 -> Bus Creator/199  "spare_199"
  Demux/228 -> Bus Creator/200  "spare_200"
